simulink model "PID"  (R2024b)
settings: Solver=FixedStepDiscrete  StartTime=0.0  StopTime=2000  RelTol=1e-3
undefined symbols (not defined in the file): DiscIntNeverNeededParam
libraries: slpidlib x1, simulink x1
settings Model: DataTypeOverride=Off  Creator=andu  LastModifiedBy=andu
settings DataIOCC: SaveOutput=off  SaveTime=off
settings OptimizationCC: BlockReduction=off  ConditionallyExecuteInputs=off  DefaultParameterBehavior=Inlined  InheritOutputTypeSmallerThanSingle=on
settings DebuggingCC: SignalRangeChecking=error  AlgebraicLoopMsg=error  SingleTaskRateTransMsg=error  IntegerOverflowMsg=none  ParameterDowncastMsg=none  ParameterOverflowMsg=none  ParameterPrecisionLossMsg=none  UnconnectedInputMsg=warning  UnconnectedOutputMsg=warning  UnconnectedLineMsg=warning  IntegerSaturationMsg=none
settings HardwareCC: ProdBitPerPointer=32  ProdBitPerSizeT=32  ProdBitPerPtrDiffT=32  ProdLargestAtomicFloat=None  ProdIntDivRoundTo=Undefined  ProdEndianess=Unspecified  ProdWordSize=32  ProdHWDeviceType=ASIC/FPGA->ASIC/FPGA  TargetBitPerLong=64  TargetBitPerPointer=64  TargetBitPerSizeT=64  TargetBitPerPtrDiffT=64  TargetLongLongMode=on  TargetIntDivRoundTo=Zero  TargetEndianess=LittleEndian  TargetWordSize=64  TargetHWDeviceType=Custom Processor->MATLAB Host Computer  ProdEqTarget=off

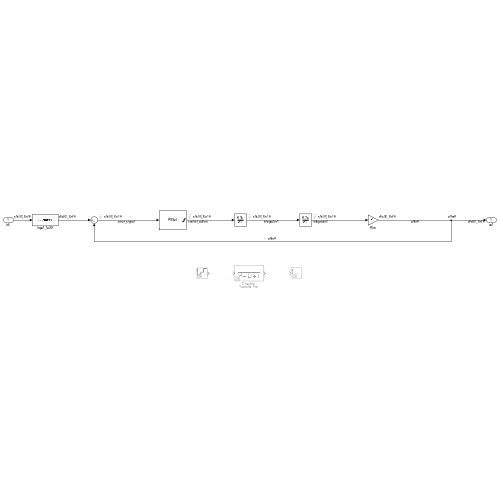
[thumbnail: Simulink's stored preview of the top-level diagram]
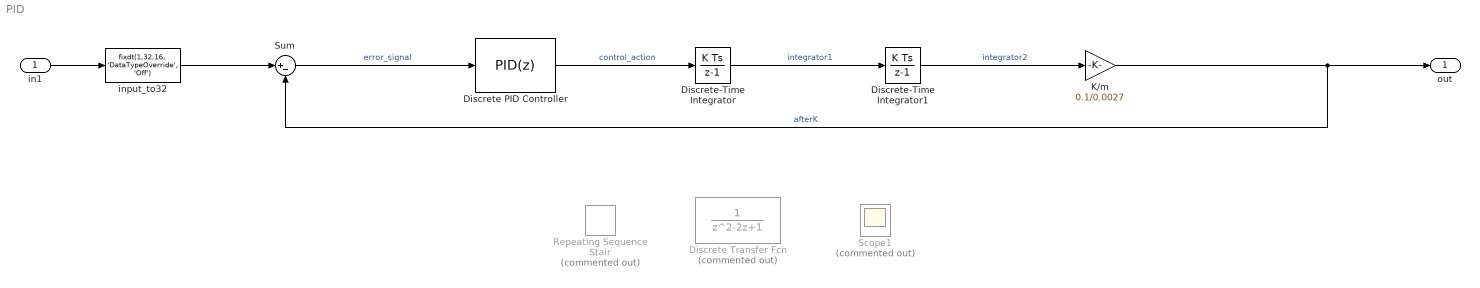
== system PID ==
  in1 : Inport
  Discrete Transfer Fcn : DiscreteTransferFcn  Commented=on  Denominator=[1 -2 1]  InitialStates=2  a0EqualsOne=on  NumCoefMin=0  NumCoefMax=4095  DenCoefMin=0  DenCoefMax=4095  OutMin=0  OutMax=4095  StateDataTypeStr=fixdt(1,16,0, 'DataTypeOverride', 'Off')  NumCoefDataTypeStr=fixdt(1,16,0, 'DataTypeOverride', 'Off')  DenCoefDataTypeStr=fixdt(1,16,0, 'DataTypeOverride', 'Off')  NumProductDataTypeStr=fixdt(1,16,0, 'DataTypeOverride', 'Off')  DenProductDataTypeStr=fixdt(1,16,-2, 'DataTypeOverride', 'Off')  NumAccumDataTypeStr=fixdt(1,16,0, 'DataTypeOverride', 'Off')  DenAccumDataTypeStr=fixdt(1,16,0, 'DataTypeOverride', 'Off')  OutDataTypeStr=fixdt(1,16,0, 'DataTypeOverride', 'Off')
  Discrete PID Controller : slpidlib/PID Controller  Controller=PID  Form=Parallel  TimeDomain=Discrete-time  UseExternalTs=off  SampleTime=0.0078125  IntegratorMethod=Forward Euler  FilterMethod=Forward Euler  ControllerParametersSource=internal  P=6.68437480474219e-05  I=0.000001  UseKiTs=off  D=0.01  UseExternalDerivativeSource=off  N=100  UseFilter=on  TunerSelectOption=Frequency Response Based  ZeroCross=off  InitialConditionSource=internal  InitialConditionForIntegrator=0  InitialConditionForFilter=0  DifferentiatorICPrevScaledInput=0  ExternalReset=none  TrackingMode=off  Kt=1  LimitOutput=on  SatLimitsSource=internal  UpperSaturationLimit=4095  LowerSaturationLimit=-4095  LinearizeAsGain=on  AntiWindupMode=clamping  Kb=1  LimitIntegrator=on  UpperIntegratorSaturationLimit=100  LowerIntegratorSaturationLimit=-100  SaturateOnIntegerOverflow=on  PGainOutDataTypeStr=fixdt(1,32,16, 'DataTypeOverride', 'Off')  PProdOutDataTypeStr=fixdt(1,32,16, 'DataTypeOverride', 'Off')  POutMin=-1000  POutMax=1000  IGainOutDataTypeStr=fixdt(1,32,16, 'DataTypeOverride', 'Off')  IProdOutDataTypeStr=fixdt(1,32,16, 'DataTypeOverride', 'Off')  IOutMin=-1000  IOutMax=1000  DGainOutDataTypeStr=fixdt(1,32,16, 'DataTypeOverride', 'Off')  DProdOutDataTypeStr=fixdt(1,32,16, 'DataTypeOverride', 'Off')  DOutMin=-1000  DOutMax=1000  NGainOutDataTypeStr=fixdt(1,32,16, 'DataTypeOverride', 'Off')  NProdOutDataTypeStr=fixdt(1,32,16, 'DataTypeOverride', 'Off')  NOutMin=[]  NOutMax=[]  SumOutDataTypeStr=fixdt(1,32,16, 'DataTypeOverride', 'Off')  SumOutMin=-4095  SumOutMax=4095  SaturationOutDataTypeStr=fixdt(1,32,16, 'DataTypeOverride', 'Off')  SaturationOutMin=-4095  SaturationOutMax=4095  PParamDataTypeStr=fixdt(1,32,16, 'DataTypeOverride', 'Off')  PParamMin=-100  PParamMax=100  IParamDataTypeStr=fixdt(1,32,16, 'DataTypeOverride', 'Off')  IParamMin=-100  IParamMax=100  DParamDataTypeStr=fixdt(1,32,16, 'DataTypeOverride', 'Off')  DParamMin=-100  DParamMax=100  NParamDataTypeStr=fixdt(1,32,16, 'DataTypeOverride', 'Off')  NParamMin=[]  NParamMax=[]  KbParamMin=[]  KbParamMax=[]  KtParamMin=[]  KtParamMax=[]  KbOutMin=[]  KbOutMax=[]  KtOutMin=[]  KtOutMax=[]  IntegratorOutDataTypeStr=fixdt(1,32,16, 'DataTypeOverride', 'Off')  IntegratorOutMin=-100  IntegratorOutMax=100  FilterOutDataTypeStr=fixdt(1,32,16, 'DataTypeOverride', 'Off')  FilterOutMin=[]  FilterOutMax=[]  SumI1OutMin=[]  SumI1OutMax=[]  SumI2OutMin=[]  SumI2OutMax=[]  SumI3OutMin=[]  SumI3OutMax=[]  SumI4OutMin=[]  SumI4OutMax=[]  SumDOutDataTypeStr=fixdt(1,32,16, 'DataTypeOverride', 'Off')  SumDOutMin=[]  SumDOutMax=[]  SumAccumDataTypeStr=fixdt(1,32,16, 'DataTypeOverride', 'Off')  SumDAccumDataTypeStr=fixdt(1,32,16, 'DataTypeOverride', 'Off')  DifferentiatorOutDataTypeStr=fixdt(1,32,16, 'DataTypeOverride', 'Off')  DifferentiatorOutMin=-100  DifferentiatorOutMax=100  FilterDiffNumProductOutputDataTypeStr=fixdt(1,32,16, 'DataTypeOverride', 'Off')  FilterDiffDenProductOutputDataTypeStr=fixdt(1,32,16, 'DataTypeOverride', 'Off')  FilterDiffNumAccumDataTypeStr=fixdt(1,32,16, 'DataTypeOverride', 'Off')  FilterDiffDenAccumDataTypeStr=fixdt(1,32,16, 'DataTypeOverride', 'Off')  FilterDiffOutCoefDataTypeStr=fixdt(1,32,16, 'DataTypeOverride', 'Off')  FilterDiffOutCoefMin=[]  FilterDiffOutCoefMax=[]  ReciprocalOutDataTypeStr=fixdt(1,32,16, 'DataTypeOverride', 'Off')  ReciprocalOutMin=[]  ReciprocalOutMax=[]  SumDenOutDataTypeStr=fixdt(1,32,16, 'DataTypeOverride', 'Off')  SumDenOutMin=[]  SumDenOutMax=[]  SumNumOutMin=[]  SumNumOutMax=[]  SumDenAccumDataTypeStr=fixdt(1,32,16, 'DataTypeOverride', 'Off')  DivideOutMin=[]  DivideOutMax=[]  UdiffTsProdOutMin=[]  UdiffTsProdOutMax=[]  NTsProdOutMin=[]  NTsProdOutMax=[]  UintegralTsProdOutMin=[]  UintegralTsProdOutMax=[]  UngainTsProdOutMin=[]  UngainTsProdOutMax=[]  ClampingZeroOutDataTypeStr=fixdt(1,32,16, 'DataTypeOverride', 'Off')  ClampingZeroOutMin=-100  ClampingZeroOutMax=100  FilterDenConstantOutDataTypeStr=fixdt(1,32,16, 'DataTypeOverride', 'Off')  FilterDenConstantOutMin=[]  FilterDenConstantOutMax=[]  PCopyOutDataTypeStr=Inherit: Inherit via back propagation  PCopyOutMin=[]  PCopyOutMax=[]  NCopyOutDataTypeStr=fixdt(1,32,16, 'DataTypeOverride', 'Off')  NCopyOutMin=[]  NCopyOutMax=[]  IntegratorContinuousStateAttributes=''  IntegratorStateMustResolveToSignalObject=off  IntegratorRTWStateStorageClass=Auto  FilterContinuousStateAttributes=''  FilterStateMustResolveToSignalObject=off  FilterRTWStateStorageClass=Auto  ParallelPVariant=InternalParameters  IdealPVariant=Disabled  IVariant=InternalParameters  DVariant=InternalParameters  IntegratorVariant=Discrete  SatVariant=Enabled  AWVariant=DiscClampingParallel  PCopyVariant=Disabled  TRVariant=Disabled  FdbkBlocksVariant=Forward  IdealPFdbkVariant=Disabled  SatFdbkVariant=Disabled  DerivativeFilterVariant=ForwardEulerFilter  NVariant=InternalParameters  NCopyVariant=Disabled  FilterICVariant=InternalICsFilter  IntegratorICVariant=InternalICs  ExternalResetVariant=Disabled  TRSumVariant=Passthrough  SumFdbkVariant=Disabled  SumVariant=Sum_PID  TsampFilterVariant=InternalTs  TsampNgainVariant=Passthrough  TsampIntegralVariant=Disabled_SignalSpec  ExternalSaturationOutDataTypeStr=Inherit: Same as second input  DerivativeSourceVariant=ErrorSignal  PreIntVariant=InternalPreInt
      settings: LibrarySourceBlock=|
      | hdlsllib/HDL Floating Point
      | Operations/Discrete PID Controller
  Discrete-Time Integrator : DiscreteIntegrator  SampleTime=0.0078125  OutMin=-4095  OutMax=4095  OutDataTypeStr=fixdt(1,32,16, 'DataTypeOverride', 'Off')  ICPrevOutput=DiscIntNeverNeededParam  ICPrevScaledInput=DiscIntNeverNeededParam
  Discrete-Time Integrator1 : DiscreteIntegrator  SampleTime=0.0078125  OutMin=-4095  OutMax=4095  OutDataTypeStr=fixdt(1,32,16, 'DataTypeOverride', 'Off')  ICPrevOutput=DiscIntNeverNeededParam  ICPrevScaledInput=DiscIntNeverNeededParam
  K/m : Gain  Gain=0.1/0.0027  ParamDataTypeStr=fixdt(1,32,16, 'DataTypeOverride', 'Off')  OutDataTypeStr=fixdt(1,32,16, 'DataTypeOverride', 'Off')
  Repeating Sequence Stair : simulink/Sources/Repeating Sequence Stair  Commented=on  OutValues=[100 500 1000].'  tsamp=0.0078125  OutMin=[]  OutMax=[]  OutDataTypeStr=fixdt(1,16,-2, 'DataTypeOverride', 'Off')  OutputDataTypeScalingMode=Specify via dialog  OutDataType=fixdt(1,16,-2, 'DataTypeOverride', 'Off')  ConRadixGroup=Best Precision: Vector-wise  OutScaling=[]
      settings: LibrarySourceBlock=|
      | hdlsllib/Sources/Repeating
      | Sequence
      | Stair
  Scope1 : Scope  Commented=on
  Sum : Sum  Inputs=|+-  OutDataTypeStr=fixdt(1,32,16, 'DataTypeOverride', 'Off')  AccumDataTypeStr=fixdt(1,32,16, 'DataTypeOverride', 'Off')
  input_to32 : DataTypeConversion  OutDataTypeStr=fixdt(1,32,16, 'DataTypeOverride', 'Off')  SaturateOnIntegerOverflow=off  RndMeth=Floor
  out : Outport  OutDataTypeStr=fixdt(1,32,16, 'DataTypeOverride', 'Off')
  wires:
  Sum/1 -> Discrete PID Controller/1  "error_signal"
  Discrete-Time Integrator/1 -> Discrete-Time Integrator1/1  "integrator1"
  Discrete PID Controller/1 -> Discrete-Time Integrator/1  "control_action"
  Discrete-Time Integrator1/1 -> K/m/1  "integrator2"
  K/m/1 -> out/1, Sum/2  "afterK"
  in1/1 -> input_to32/1
  input_to32/1 -> Sum/1
